simulink library "ECE1718_cnn_original"  (R2022b)
settings: Solver=VariableStepAuto  StartTime=0.0  StopTime=10.0  RelTol=1e-3
libraries: $bdroot x2
(part 2 of 2)

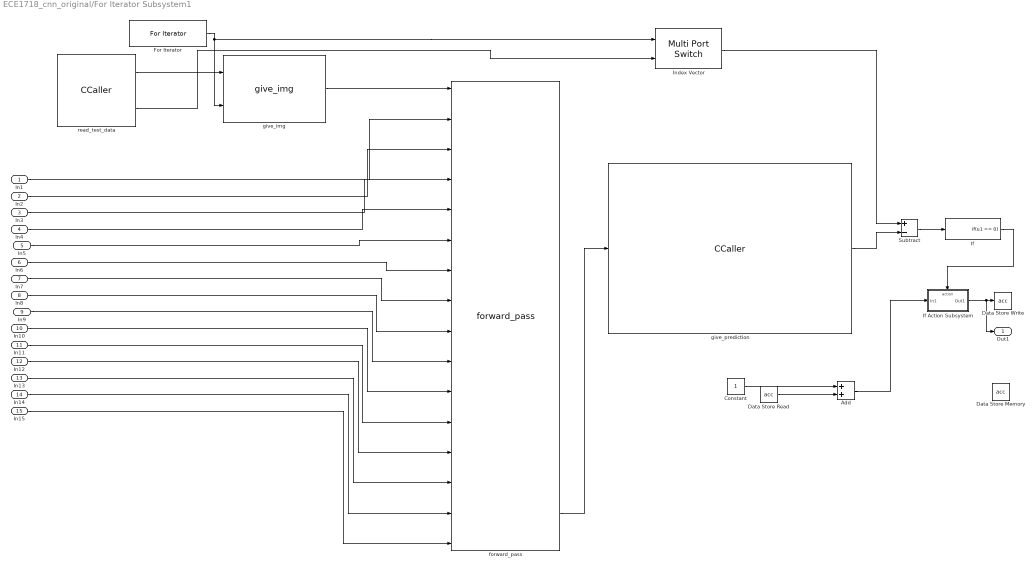
== system ECE1718_cnn_original/For Iterator Subsystem1 ==
  In1 : Inport
  In2 : Inport  Port=2
  In3 : Inport  Port=3
  In4 : Inport  Port=4
  In5 : Inport  Port=5
  In6 : Inport  Port=6
  In7 : Inport  Port=7
  In8 : Inport  Port=8
  In9 : Inport  Port=9
  In10 : Inport  Port=10
  In11 : Inport  Port=11
  In12 : Inport  Port=12
  In13 : Inport  Port=13
  In14 : Inport  Port=14
  In15 : Inport  Port=15
  Add : Sum
  Constant : Constant
  Data Store Memory : DataStoreMemory  DataStoreName=acc  WriteAfterWriteMsg=warning  ShowAdditionalParam=off
  Data Store Read : DataStoreRead  DataStoreName=acc  IndexOptions=Index vector (dialog)  Indices=1  OutputSizes=1
  Data Store Write : DataStoreWrite  DataStoreName=acc  IndexOptions=Index vector (dialog)  Indices=1  OutputSizes=1
  For Iterator : ForIterator  IterationLimit=600  IndexMode=Zero-based  IterationVariableDataType=double
  If : If  IfExpression=u1 == 0  ShowElse=off
  If Action Subsystem : Subsystem  TreatAsAtomicUnit=on
  Index Vector : MultiPortSwitch  DataPortOrder=Zero-based contiguous  Inputs=1  zeroidx=on  SaturateOnIntegerOverflow=off  InputSameDT=off
  Subtract : Sum  Inputs=+-
  forward_pass : $bdroot/For Iterator Subsystem/forward_pass  SampleTime=-1
  give_img : $bdroot/For Iterator Subsystem/give_img  SampleTime=-1
  give_prediction : CCaller  FunctionName=give_prediction  PortSpecificationStruct="%)30     .    V ,   8    (     @         %    \"     (    !     0         %  0 \"0    $    _    07)G3F%M90  4&]R=$YA;64 4V-O<&4     26YD97@     5'EP90      4VEZ90      27-';&]B86P   X    P    !@    @    $          4    (     0    ,    !         !   P!O=70 #@   #     &    \"     0         !0    @    !     P    $         $  # &]U=  .    .     8    (    !          %    \"     $    &     0         0    !@   $]U='!U=   #@   #@    &    \"     8         !0    @    !     0    $         \"0    @               X    X    !@    @    $          4    (     0    4    !         !     %    :6YT,S(    .    ,     8    (    !          %    \"     $    !     0         0  $ ,0    X    P    !@    @    ) @        4    (     0    $    !          (  0      #@   $     &    \"     0         !0    @    !    #0    $         $     T   !D96YS95]S;V9T;6%X    #@   $     &    \"     0         !0    @    !    #0    $         $     T   !D96YS95]S;V9T;6%X    #@   #@    &    \"     0         !0    @    !    !0    $         $     4   !);G!U=     X    X    !@    @    &          4    (     0    $    !          D    (               .    .     8    (    !          %    \"     $    &     0         0    !@   &1O=6)L90  #@   #     &    \"     0         !0    @    !     @    $         $  \" #$P   .    ,     8    (    \"0(        %    \"     $    !     0         \"  $"
  read_test_data : CCaller  FunctionName=read_test_data  PortSpecificationStruct="%)30     .    \" 0   8    (     @         %    \"     (    !     0         %  0 \"0    $    _    07)G3F%M90  4&]R=$YA;64 4V-O<&4     26YD97@     5'EP90      4VEZ90      27-';&]B86P   X   !     !@    @    $          4    (     0    D    !         !     )    9&%T85]T97-T          X   !     !@    @    $          4    (     0    D    !         !     )    9&%T85]T97-T          X    X    !@    @    $          4    (     0    8    !         !     &    3W5T<'5T   .    .     8    (    !@         %    \"     $    !     0         )    \"               #@   #@    &    \"     0         !0    @    !    !0    $         $     4   !U:6YT.     X    X    !@    @    $          4    (     0    <    !         !     '    -S@T,# P,  .    ,     8    (    \"0(        %    \"     $    !     0         \"  $       X   !     !@    @    $          4    (     0    H    !         !     *    ;&%B96Q?=&5S=         X   !     !@    @    $          4    (     0    H    !         !     *    ;&%B96Q?=&5S=         X    X    !@    @    $          4    (     0    8    !         !     &    3W5T<'5T   .    .     8    (    !@         %    \"     $    !     0         )    \"            / _#@   #@    &    \"     0         !0    @    !    !0    $         $     4   !U:6YT.     X    X    !@    @    $          4    (     0    4    !         !     %    ,3 P,#     .    ,     8    (    \"0(        %    \"     $    !     0         \"  $"
  Out1 : Outport
  wires:
  forward_pass/15 -> give_prediction/1
  In4/1 -> forward_pass/5
  In14/1 -> forward_pass/15
  In11/1 -> forward_pass/12
  In15/1 -> forward_pass/16
  In10/1 -> forward_pass/11
  In2/1 -> forward_pass/3
  In13/1 -> forward_pass/14
  In5/1 -> forward_pass/6
  read_test_data/1 -> give_img/1
  In3/1 -> forward_pass/4
  In12/1 -> forward_pass/13
  give_img/1 -> forward_pass/1
  In7/1 -> forward_pass/8
  In9/1 -> forward_pass/10
  In6/1 -> forward_pass/7
  In8/1 -> forward_pass/9
  In1/1 -> forward_pass/2
  For Iterator/1 -> Index Vector/1, give_img/2
  Subtract/1 -> If/1
  give_prediction/1 -> Subtract/2
  read_test_data/2 -> Index Vector/2
  Index Vector/1 -> Subtract/1
  If/1 -> If Action Subsystem/Action
  Add/1 -> If Action Subsystem/1(In1)
  If Action Subsystem/1(Out1) -> Out1/1, Data Store Write/1
  Data Store Read/1 -> Add/2
  Constant/1 -> Add/1

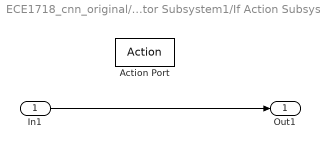
== system ECE1718_cnn_original/For Iterator Subsystem1/If Action Subsystem ==
  In1 : Inport
  Action Port : ActionPort  ActionPortLabel=if(u1 == 0)
  Out1 : Outport
  wires:
  In1/1 -> Out1/1
